simulink model "three_ringnetwork_with_control"  (R2016a)
settings: Solver=VariableStepAuto  StartTime=0.0  StopTime=0.2  RelTol=1e-3
undefined symbols (not defined in the file): vc0d
libraries: simulink x18, powerlib_meascontrol x3
(part 2 of 3)

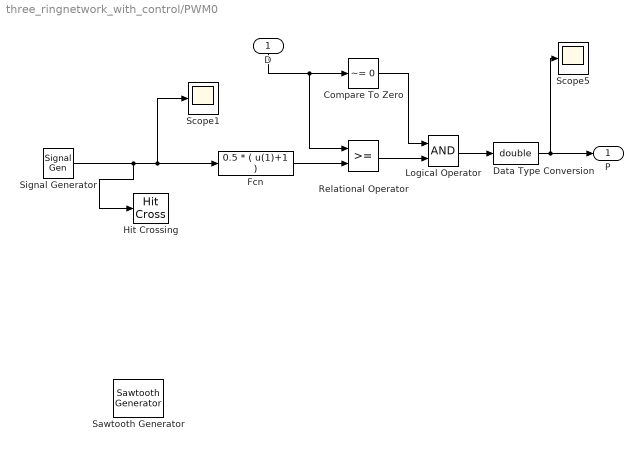
== system three_ringnetwork_with_control/PWM0 ==
  D : Inport
  Compare To Zero : simulink/Logic and Bit Operations/Compare To Zero  relop=~=  OutDataTypeStr=boolean
  Data Type Conversion : DataTypeConversion  OutMin=[0]  OutMax=[1]  OutDataTypeStr=double
  Fcn : Fcn  Expr=0.5 * ( u(1)+1 )
  Hit Crossing : HitCross  ShowOutputPort=off
  Logical Operator : Logic  AllPortsSameDT=off  OutDataTypeStr=boolean
  Relational Operator : RelationalOperator  OutDataTypeStr=boolean
  Sawtooth Generator : powerlib_meascontrol/Pulse & Signal Generators/Sawtooth Generator  Freq=1e3  Phase=180  Ts=0
  Scope1 : Scope
  Scope5 : Scope
  Signal Generator : SignalGenerator  WaveForm=sawtooth  Frequency=10000
  P : Outport
  wires:
  Logical Operator/1 -> Data Type Conversion/1
  Relational Operator/1 -> Logical Operator/2
  Fcn/1 -> Relational Operator/2
  D/1 -> Relational Operator/1, Compare To Zero/1
  Data Type Conversion/1 -> P/1, Scope5/1
  Compare To Zero/1 -> Logical Operator/1
  Signal Generator/1 -> Hit Crossing/1, Scope1/1, Fcn/1

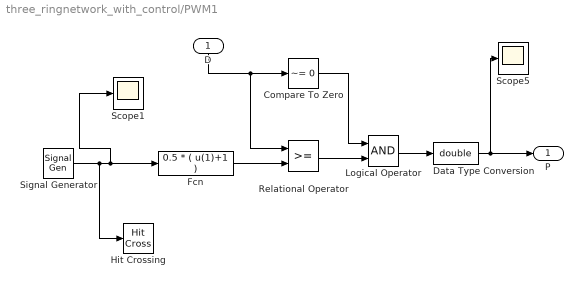
== system three_ringnetwork_with_control/PWM1 ==
  D : Inport
  Compare To Zero : simulink/Logic and Bit Operations/Compare To Zero  relop=~=  OutDataTypeStr=boolean
  Data Type Conversion : DataTypeConversion  OutDataTypeStr=double
  Fcn : Fcn  Expr=0.5 * ( u(1)+1 )
  Hit Crossing : HitCross
  Logical Operator : Logic  AllPortsSameDT=off  OutDataTypeStr=boolean
  Relational Operator : RelationalOperator  OutDataTypeStr=boolean
  Scope1 : Scope
  Scope5 : Scope
  Signal Generator : SignalGenerator  WaveForm=sawtooth  Frequency=10000
  P : Outport
  wires:
  Logical Operator/1 -> Data Type Conversion/1
  Relational Operator/1 -> Logical Operator/2
  Signal Generator/1 -> Hit Crossing/1, Scope1/1, Fcn/1
  Fcn/1 -> Relational Operator/2
  D/1 -> Relational Operator/1, Compare To Zero/1
  Data Type Conversion/1 -> P/1, Scope5/1
  Compare To Zero/1 -> Logical Operator/1

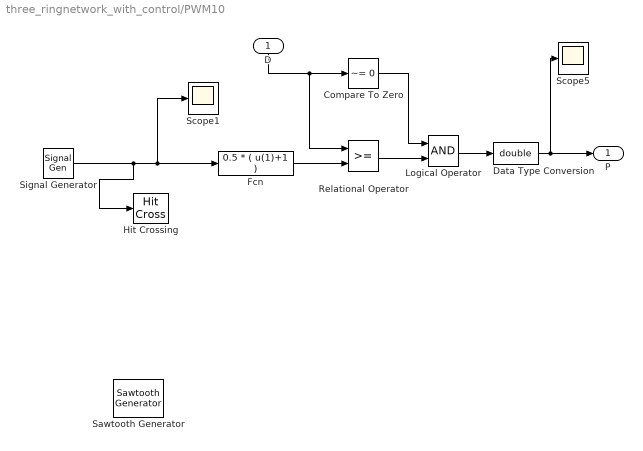
== system three_ringnetwork_with_control/PWM10 ==
  D : Inport
  Compare To Zero : simulink/Logic and Bit Operations/Compare To Zero  relop=~=  OutDataTypeStr=boolean  ZeroCross=off
  Data Type Conversion : DataTypeConversion  OutMin=[0]  OutMax=[1]  OutDataTypeStr=double
  Fcn : Fcn  Expr=0.5 * ( u(1)+1 )
  Hit Crossing : HitCross  ShowOutputPort=off
  Logical Operator : Logic  AllPortsSameDT=off  OutDataTypeStr=boolean
  Relational Operator : RelationalOperator  OutDataTypeStr=boolean  ZeroCross=off
  Sawtooth Generator : powerlib_meascontrol/Pulse & Signal Generators/Sawtooth Generator  Freq=1e3  Phase=180  Ts=0
  Scope1 : Scope
  Scope5 : Scope
  Signal Generator : SignalGenerator  WaveForm=sawtooth  Frequency=10000
  P : Outport
  wires:
  Logical Operator/1 -> Data Type Conversion/1
  Relational Operator/1 -> Logical Operator/2
  Fcn/1 -> Relational Operator/2
  D/1 -> Relational Operator/1, Compare To Zero/1
  Data Type Conversion/1 -> P/1, Scope5/1
  Compare To Zero/1 -> Logical Operator/1
  Signal Generator/1 -> Hit Crossing/1, Scope1/1, Fcn/1

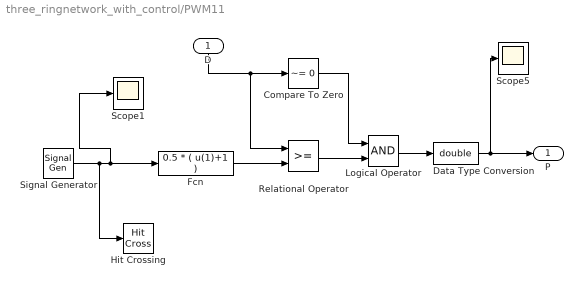
== system three_ringnetwork_with_control/PWM11 ==
  D : Inport
  Compare To Zero : simulink/Logic and Bit Operations/Compare To Zero  relop=~=  OutDataTypeStr=boolean
  Data Type Conversion : DataTypeConversion  OutDataTypeStr=double
  Fcn : Fcn  Expr=0.5 * ( u(1)+1 )
  Hit Crossing : HitCross
  Logical Operator : Logic  AllPortsSameDT=off  OutDataTypeStr=boolean
  Relational Operator : RelationalOperator  OutDataTypeStr=boolean
  Scope1 : Scope
  Scope5 : Scope
  Signal Generator : SignalGenerator  WaveForm=sawtooth  Frequency=10000
  P : Outport
  wires:
  Logical Operator/1 -> Data Type Conversion/1
  Relational Operator/1 -> Logical Operator/2
  Signal Generator/1 -> Hit Crossing/1, Scope1/1, Fcn/1
  Fcn/1 -> Relational Operator/2
  D/1 -> Relational Operator/1, Compare To Zero/1
  Data Type Conversion/1 -> P/1, Scope5/1
  Compare To Zero/1 -> Logical Operator/1

== system three_ringnetwork_with_control/PWM12 ==
  D : Inport
  Compare To Zero : simulink/Logic and Bit Operations/Compare To Zero  relop=~=  OutDataTypeStr=boolean
  Data Type Conversion : DataTypeConversion  OutDataTypeStr=double
  Fcn : Fcn  Expr=0.5 * ( u(1)+1 )
  Hit Crossing : HitCross
  Logical Operator : Logic  AllPortsSameDT=off  OutDataTypeStr=boolean
  Relational Operator : RelationalOperator  OutDataTypeStr=boolean
  Scope1 : Scope
  Scope5 : Scope
  Signal Generator : SignalGenerator  WaveForm=sawtooth  Frequency=10000
  P : Outport
  wires:
  Logical Operator/1 -> Data Type Conversion/1
  Relational Operator/1 -> Logical Operator/2
  Signal Generator/1 -> Hit Crossing/1, Scope1/1, Fcn/1
  Fcn/1 -> Relational Operator/2
  D/1 -> Relational Operator/1, Compare To Zero/1
  Data Type Conversion/1 -> P/1, Scope5/1
  Compare To Zero/1 -> Logical Operator/1

== system three_ringnetwork_with_control/PWM13 ==
  D : Inport
  Compare To Zero : simulink/Logic and Bit Operations/Compare To Zero  relop=~=  OutDataTypeStr=boolean
  Data Type Conversion : DataTypeConversion  OutDataTypeStr=double
  Fcn : Fcn  Expr=0.5 * ( u(1)+1 )
  Hit Crossing : HitCross
  Logical Operator : Logic  AllPortsSameDT=off  OutDataTypeStr=boolean
  Relational Operator : RelationalOperator  OutDataTypeStr=boolean
  Scope1 : Scope
  Scope5 : Scope
  Signal Generator : SignalGenerator  WaveForm=sawtooth  Frequency=10000
  P : Outport
  wires:
  Logical Operator/1 -> Data Type Conversion/1
  Relational Operator/1 -> Logical Operator/2
  Signal Generator/1 -> Scope1/1, Hit Crossing/1, Fcn/1
  Fcn/1 -> Relational Operator/2
  D/1 -> Relational Operator/1, Compare To Zero/1
  Data Type Conversion/1 -> P/1, Scope5/1
  Compare To Zero/1 -> Logical Operator/1

== system three_ringnetwork_with_control/PWM14 ==
  D : Inport
  Compare To Zero : simulink/Logic and Bit Operations/Compare To Zero  relop=~=  OutDataTypeStr=boolean
  Data Type Conversion : DataTypeConversion  OutDataTypeStr=double
  Fcn : Fcn  Expr=0.5 * ( u(1)+1 )
  Hit Crossing : HitCross
  Logical Operator : Logic  AllPortsSameDT=off  OutDataTypeStr=boolean
  Relational Operator : RelationalOperator  OutDataTypeStr=boolean
  Scope5 : Scope
  Signal Generator : SignalGenerator  WaveForm=sawtooth  Frequency=10000
  P : Outport
  wires:
  Logical Operator/1 -> Data Type Conversion/1
  Relational Operator/1 -> Logical Operator/2
  Signal Generator/1 -> Hit Crossing/1, Fcn/1
  Fcn/1 -> Relational Operator/2
  D/1 -> Relational Operator/1, Compare To Zero/1
  Data Type Conversion/1 -> P/1, Scope5/1
  Compare To Zero/1 -> Logical Operator/1

== system three_ringnetwork_with_control/PWM2 ==
  D : Inport
  Compare To Zero : simulink/Logic and Bit Operations/Compare To Zero  relop=~=  OutDataTypeStr=boolean
  Data Type Conversion : DataTypeConversion  OutDataTypeStr=double
  Fcn : Fcn  Expr=0.5 * ( u(1)+1 )
  Hit Crossing : HitCross
  Logical Operator : Logic  AllPortsSameDT=off  OutDataTypeStr=boolean
  Relational Operator : RelationalOperator  OutDataTypeStr=boolean
  Scope1 : Scope
  Scope5 : Scope
  Signal Generator : SignalGenerator  WaveForm=sawtooth  Frequency=10000
  P : Outport
  wires:
  Logical Operator/1 -> Data Type Conversion/1
  Relational Operator/1 -> Logical Operator/2
  Signal Generator/1 -> Hit Crossing/1, Scope1/1, Fcn/1
  Fcn/1 -> Relational Operator/2
  D/1 -> Relational Operator/1, Compare To Zero/1
  Data Type Conversion/1 -> P/1, Scope5/1
  Compare To Zero/1 -> Logical Operator/1

== system three_ringnetwork_with_control/PWM3 ==
  D : Inport
  Compare To Zero : simulink/Logic and Bit Operations/Compare To Zero  relop=~=  OutDataTypeStr=boolean
  Data Type Conversion : DataTypeConversion  OutDataTypeStr=double
  Fcn : Fcn  Expr=0.5 * ( u(1)+1 )
  Hit Crossing : HitCross
  Logical Operator : Logic  AllPortsSameDT=off  OutDataTypeStr=boolean
  Relational Operator : RelationalOperator  OutDataTypeStr=boolean
  Scope1 : Scope
  Scope5 : Scope
  Signal Generator : SignalGenerator  WaveForm=sawtooth  Frequency=10000
  P : Outport
  wires:
  Logical Operator/1 -> Data Type Conversion/1
  Relational Operator/1 -> Logical Operator/2
  Signal Generator/1 -> Scope1/1, Hit Crossing/1, Fcn/1
  Fcn/1 -> Relational Operator/2
  D/1 -> Relational Operator/1, Compare To Zero/1
  Data Type Conversion/1 -> P/1, Scope5/1
  Compare To Zero/1 -> Logical Operator/1

== system three_ringnetwork_with_control/PWM4 ==
  D : Inport
  Compare To Zero : simulink/Logic and Bit Operations/Compare To Zero  relop=~=  OutDataTypeStr=boolean
  Data Type Conversion : DataTypeConversion  OutDataTypeStr=double
  Fcn : Fcn  Expr=0.5 * ( u(1)+1 )
  Hit Crossing : HitCross
  Logical Operator : Logic  AllPortsSameDT=off  OutDataTypeStr=boolean
  Relational Operator : RelationalOperator  OutDataTypeStr=boolean
  Scope5 : Scope
  Signal Generator : SignalGenerator  WaveForm=sawtooth  Frequency=10000
  P : Outport
  wires:
  Logical Operator/1 -> Data Type Conversion/1
  Relational Operator/1 -> Logical Operator/2
  Signal Generator/1 -> Hit Crossing/1, Fcn/1
  Fcn/1 -> Relational Operator/2
  D/1 -> Relational Operator/1, Compare To Zero/1
  Data Type Conversion/1 -> P/1, Scope5/1
  Compare To Zero/1 -> Logical Operator/1

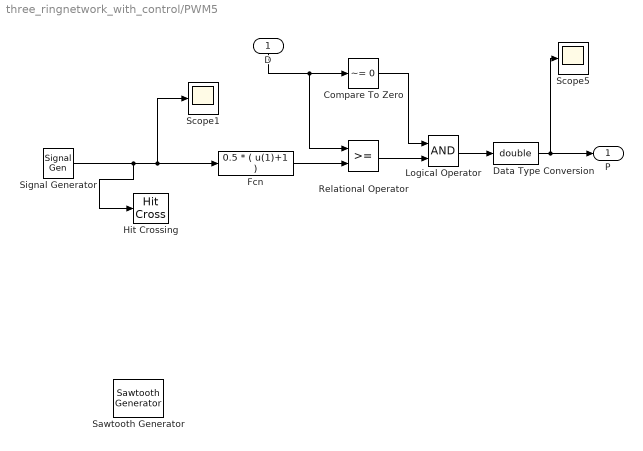
== system three_ringnetwork_with_control/PWM5 ==
  D : Inport
  Compare To Zero : simulink/Logic and Bit Operations/Compare To Zero  relop=~=  OutDataTypeStr=boolean
  Data Type Conversion : DataTypeConversion  OutMin=[0]  OutMax=[1]  OutDataTypeStr=double
  Fcn : Fcn  Expr=0.5 * ( u(1)+1 )
  Hit Crossing : HitCross  ShowOutputPort=off
  Logical Operator : Logic  AllPortsSameDT=off  OutDataTypeStr=boolean
  Relational Operator : RelationalOperator  OutDataTypeStr=boolean
  Sawtooth Generator : powerlib_meascontrol/Pulse & Signal Generators/Sawtooth Generator  Freq=1e3  Phase=180  Ts=0
  Scope1 : Scope
  Scope5 : Scope
  Signal Generator : SignalGenerator  WaveForm=sawtooth  Frequency=10000
  P : Outport
  wires:
  Logical Operator/1 -> Data Type Conversion/1
  Relational Operator/1 -> Logical Operator/2
  Fcn/1 -> Relational Operator/2
  D/1 -> Relational Operator/1, Compare To Zero/1
  Data Type Conversion/1 -> P/1, Scope5/1
  Compare To Zero/1 -> Logical Operator/1
  Signal Generator/1 -> Hit Crossing/1, Scope1/1, Fcn/1

== system three_ringnetwork_with_control/PWM6 ==
  D : Inport
  Compare To Zero : simulink/Logic and Bit Operations/Compare To Zero  relop=~=  OutDataTypeStr=boolean
  Data Type Conversion : DataTypeConversion  OutDataTypeStr=double
  Fcn : Fcn  Expr=0.5 * ( u(1)+1 )
  Hit Crossing : HitCross
  Logical Operator : Logic  AllPortsSameDT=off  OutDataTypeStr=boolean
  Relational Operator : RelationalOperator  OutDataTypeStr=boolean
  Scope1 : Scope
  Scope5 : Scope
  Signal Generator : SignalGenerator  WaveForm=sawtooth  Frequency=10000
  P : Outport
  wires:
  Logical Operator/1 -> Data Type Conversion/1
  Relational Operator/1 -> Logical Operator/2
  Signal Generator/1 -> Hit Crossing/1, Scope1/1, Fcn/1
  Fcn/1 -> Relational Operator/2
  D/1 -> Relational Operator/1, Compare To Zero/1
  Data Type Conversion/1 -> P/1, Scope5/1
  Compare To Zero/1 -> Logical Operator/1

== system three_ringnetwork_with_control/PWM7 ==
  D : Inport
  Compare To Zero : simulink/Logic and Bit Operations/Compare To Zero  relop=~=  OutDataTypeStr=boolean
  Data Type Conversion : DataTypeConversion  OutDataTypeStr=double
  Fcn : Fcn  Expr=0.5 * ( u(1)+1 )
  Hit Crossing : HitCross
  Logical Operator : Logic  AllPortsSameDT=off  OutDataTypeStr=boolean
  Relational Operator : RelationalOperator  OutDataTypeStr=boolean
  Scope1 : Scope
  Scope5 : Scope
  Signal Generator : SignalGenerator  WaveForm=sawtooth  Frequency=10000
  P : Outport
  wires:
  Logical Operator/1 -> Data Type Conversion/1
  Relational Operator/1 -> Logical Operator/2
  Signal Generator/1 -> Hit Crossing/1, Scope1/1, Fcn/1
  Fcn/1 -> Relational Operator/2
  D/1 -> Relational Operator/1, Compare To Zero/1
  Data Type Conversion/1 -> P/1, Scope5/1
  Compare To Zero/1 -> Logical Operator/1

== system three_ringnetwork_with_control/PWM8 ==
  D : Inport
  Compare To Zero : simulink/Logic and Bit Operations/Compare To Zero  relop=~=  OutDataTypeStr=boolean
  Data Type Conversion : DataTypeConversion  OutDataTypeStr=double
  Fcn : Fcn  Expr=0.5 * ( u(1)+1 )
  Hit Crossing : HitCross
  Logical Operator : Logic  AllPortsSameDT=off  OutDataTypeStr=boolean
  Relational Operator : RelationalOperator  OutDataTypeStr=boolean
  Scope1 : Scope
  Scope5 : Scope
  Signal Generator : SignalGenerator  WaveForm=sawtooth  Frequency=10000
  P : Outport
  wires:
  Logical Operator/1 -> Data Type Conversion/1
  Relational Operator/1 -> Logical Operator/2
  Signal Generator/1 -> Scope1/1, Hit Crossing/1, Fcn/1
  Fcn/1 -> Relational Operator/2
  D/1 -> Relational Operator/1, Compare To Zero/1
  Data Type Conversion/1 -> P/1, Scope5/1
  Compare To Zero/1 -> Logical Operator/1

== system three_ringnetwork_with_control/PWM9 ==
  D : Inport
  Compare To Zero : simulink/Logic and Bit Operations/Compare To Zero  relop=~=  OutDataTypeStr=boolean
  Data Type Conversion : DataTypeConversion  OutDataTypeStr=double
  Fcn : Fcn  Expr=0.5 * ( u(1)+1 )
  Hit Crossing : HitCross
  Logical Operator : Logic  AllPortsSameDT=off  OutDataTypeStr=boolean
  Relational Operator : RelationalOperator  OutDataTypeStr=boolean
  Scope5 : Scope
  Signal Generator : SignalGenerator  WaveForm=sawtooth  Frequency=10000
  P : Outport
  wires:
  Logical Operator/1 -> Data Type Conversion/1
  Relational Operator/1 -> Logical Operator/2
  Signal Generator/1 -> Hit Crossing/1, Fcn/1
  Fcn/1 -> Relational Operator/2
  D/1 -> Relational Operator/1, Compare To Zero/1
  Data Type Conversion/1 -> P/1, Scope5/1
  Compare To Zero/1 -> Logical Operator/1

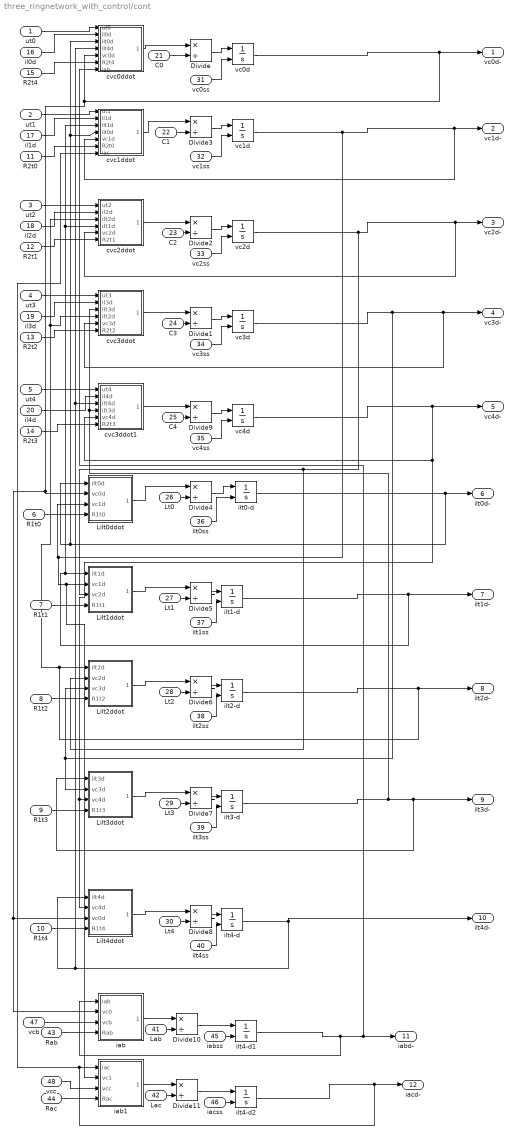
== system three_ringnetwork_with_control/cont ==
  ut0 : Inport
  ut1 : Inport  Port=2
  ut2 : Inport  Port=3
  ut3 : Inport  Port=4
  ut4 : Inport  Port=5
  R1t0 : Inport  Port=6
  R1t1 : Inport  Port=7
  R1t2 : Inport  Port=8
  R1t3 : Inport  Port=9
  R1t4 : Inport  Port=10
  R2t0 : Inport  Port=11
  R2t1 : Inport  Port=12
  R2t2 : Inport  Port=13
  R2t3 : Inport  Port=14
  R2t4 : Inport  Port=15
  il0d : Inport  Port=16
  il1d : Inport  Port=17
  il2d : Inport  Port=18
  il3d : Inport  Port=19
  il4d : Inport  Port=20
  C0 : Inport  Port=21
  C1 : Inport  Port=22
  C2 : Inport  Port=23
  C3 : Inport  Port=24
  C4 : Inport  Port=25
  Lt0 : Inport  Port=26
  Lt1 : Inport  Port=27
  Lt2 : Inport  Port=28
  Lt3 : Inport  Port=29
  Lt4 : Inport  Port=30
  vc0ss : Inport  Port=31
  vc1ss : Inport  Port=32
  vc2ss : Inport  Port=33
  vc3ss : Inport  Port=34
  vc4ss : Inport  Port=35
  ilt0ss : Inport  Port=36
  ilt1ss : Inport  Port=37
  ilt2ss : Inport  Port=38
  ilt3ss : Inport  Port=39
  ilt4ss : Inport  Port=40
  Lab : Inport  Port=41
  Lac : Inport  Port=42
  Rab : Inport  Port=43
  Rac : Inport  Port=44
  iabss : Inport  Port=45
  iacss : Inport  Port=46
  vcb : Inport  Port=47
  vcc : Inport  Port=48
  Divide{,1..11} (12 alike) : Product  Inputs=*/
  Lilt0ddot : MATLAB Function  TreatAsAtomicUnit=on
  Lilt1ddot : MATLAB Function  TreatAsAtomicUnit=on
  Lilt2ddot : MATLAB Function  TreatAsAtomicUnit=on
  Lilt3ddot : MATLAB Function  TreatAsAtomicUnit=on
  Lilt4ddot : MATLAB Function  TreatAsAtomicUnit=on
  cvc0ddot : MATLAB Function  TreatAsAtomicUnit=on
  cvc1ddot : MATLAB Function  TreatAsAtomicUnit=on
  cvc2ddot : MATLAB Function  TreatAsAtomicUnit=on
  cvc3ddot : MATLAB Function  TreatAsAtomicUnit=on
  cvc3ddot1 : MATLAB Function  TreatAsAtomicUnit=on
  iab : MATLAB Function  TreatAsAtomicUnit=on
  iab1 : MATLAB Function  TreatAsAtomicUnit=on
  ilt0-d : Integrator  InitialConditionSource=external  InitialCondition=vc0d
  ilt1-d : Integrator  InitialConditionSource=external  InitialCondition=vc0d
  ilt2-d : Integrator  InitialConditionSource=external  InitialCondition=vc0d
  ilt3-d : Integrator  InitialConditionSource=external  InitialCondition=vc0d
  ilt4-d : Integrator  InitialConditionSource=external  InitialCondition=vc0d
  ilt4-d1 : Integrator  InitialConditionSource=external  InitialCondition=vc0d
  ilt4-d2 : Integrator  InitialConditionSource=external  InitialCondition=vc0d
  vc0d : Integrator  InitialConditionSource=external  InitialCondition=vc0d
  vc1d : Integrator  InitialConditionSource=external  InitialCondition=vc0d
  vc2d : Integrator  InitialConditionSource=external  InitialCondition=vc0d
  vc3d : Integrator  InitialConditionSource=external  InitialCondition=vc0d
  vc4d : Integrator  InitialConditionSource=external  InitialCondition=vc0d
  vc0d- : Outport
  vc1d- : Outport  Port=2
  vc2d- : Outport  Port=3
  vc3d- : Outport  Port=4
  vc4d- : Outport  Port=5
  ilt0d- : Outport  Port=6
  ilt1d- : Outport  Port=7
  ilt2d- : Outport  Port=8
  ilt3d- : Outport  Port=9
  ilt4d- : Outport  Port=10
  iabd- : Outport  Port=11
  iacd- : Outport  Port=12
  wires:
  cvc0ddot/1(Cvc0ddot) -> Divide/1
  ut0/1 -> cvc0ddot/1(ut0)
  il0d/1 -> cvc0ddot/2(il0d)
  C0/1 -> Divide/2
  C1/1 -> Divide3/2
  C2/1 -> Divide2/2
  Divide3/1 -> vc1d/1
  Divide/1 -> vc0d/1
  cvc1ddot/1(Cvc1ddot) -> Divide3/1
  ut1/1 -> cvc1ddot/1(ut1)
  il1d/1 -> cvc1ddot/2(il1d)
  R2t4/1 -> cvc0ddot/6(R2t4)
  R2t0/1 -> cvc1ddot/6(R2t0)
  cvc2ddot/1(Cvc2ddot) -> Divide2/1
  ut2/1 -> cvc2ddot/1(ut2)
  il2d/1 -> cvc2ddot/2(il2d)
  R2t1/1 -> cvc2ddot/6(R2t1)
  Divide2/1 -> vc2d/1
  Divide4/1 -> ilt0-d/1
  Divide5/1 -> ilt1-d/1
  Divide6/1 -> ilt2-d/1
  Lt0/1 -> Divide4/2
  Lt1/1 -> Divide5/2
  Lt2/1 -> Divide6/2
  Lilt2ddot/1(Lilt2ddot) -> Divide6/1
  Lilt1ddot/1(Lilt1ddot) -> Divide5/1
  Lilt0ddot/1(Lilt0ddot) -> Divide4/1
  R1t1/1 -> Lilt1ddot/4(R1t1)
  R1t2/1 -> Lilt2ddot/4(R1t2)
  vc0ss/1 -> vc0d/2
  vc1ss/1 -> vc1d/2
  vc2ss/1 -> vc2d/2
  ilt0ss/1 -> ilt0-d/2
  ilt2ss/1 -> ilt2-d/2
  ilt1ss/1 -> ilt1-d/2
  R1t0/1 -> Lilt0ddot/4(R1t0)
  C3/1 -> Divide1/2
  cvc3ddot/1(Cvc3ddot) -> Divide1/1
  ut3/1 -> cvc3ddot/1(ut3)
  il3d/1 -> cvc3ddot/2(il3d)
  R2t2/1 -> cvc3ddot/6(R2t2)
  Divide1/1 -> vc3d/1
  vc3ss/1 -> vc3d/2
  Divide7/1 -> ilt3-d/1
  Lt3/1 -> Divide7/2
  Lilt3ddot/1(Lilt3ddot) -> Divide7/1
  R1t3/1 -> Lilt3ddot/4(R1t3)
  ilt3ss/1 -> ilt3-d/2
  Divide8/1 -> ilt4-d/1
  Lt4/1 -> Divide8/2
  Lilt4ddot/1(Lilt4ddot) -> Divide8/1
  R1t4/1 -> Lilt4ddot/4(R1t4)
  ilt4ss/1 -> ilt4-d/2
  C4/1 -> Divide9/2
  cvc3ddot1/1(Cvc4ddot) -> Divide9/1
  Divide9/1 -> vc4d/1
  vc4ss/1 -> vc4d/2
  vc0d/1 -> cvc0ddot/5(vc0d), iab/2(vc0), Lilt4ddot/3(vc0d), Lilt0ddot/2(vc0d), vc0d-/1
  vc1d/1 -> iab1/2(vc1), Lilt1ddot/2(vc1d), Lilt0ddot/3(vc1d), cvc1ddot/5(vc1d), vc1d-/1
  vc2d/1 -> Lilt2ddot/2(vc2d), Lilt1ddot/3(vc2d), cvc2ddot/5(vc2d), vc2d-/1
  vc3d/1 -> Lilt3ddot/2(vc3d), Lilt2ddot/3(vc3d), cvc3ddot/5(vc3d), vc3d-/1
  vc4d/1 -> cvc3ddot1/5(vc4d), Lilt4ddot/2(vc4d), Lilt3ddot/3(vc4d), vc4d-/1
  ilt0-d/1 -> cvc0ddot/3(ilt0d), cvc1ddot/4(ilt0d), Lilt0ddot/1(ilt0d), ilt0d-/1
  ilt1-d/1 -> cvc2ddot/4(ilt1d), cvc1ddot/3(ilt1d), Lilt1ddot/1(ilt1d), ilt1d-/1
  ilt2-d/1 -> Lilt2ddot/1(ilt2d), cvc3ddot/4(ilt2d), cvc2ddot/3(ilt2d), ilt2d-/1
  ilt4-d/1 -> cvc0ddot/4(ilt4d), cvc3ddot1/3(ilt4d), Lilt4ddot/1(ilt4d), ilt4d-/1
  ut4/1 -> cvc3ddot1/1(ut4)
  il4d/1 -> cvc3ddot1/2(il4d)
  R2t3/1 -> cvc3ddot1/6(R2t3)
  ilt3-d/1 -> cvc3ddot/3(ilt3d), cvc3ddot1/4(ilt3d), Lilt3ddot/1(ilt3d), ilt3d-/1
  iab/1(Labddot) -> Divide10/1
  Divide10/1 -> ilt4-d1/1
  iab1/1(Lacddot) -> Divide11/1
  Divide11/1 -> ilt4-d2/1
  ilt4-d1/1 -> iab/1(iab), cvc0ddot/7(iab), iabd-/1
  ilt4-d2/1 -> cvc1ddot/7(iac), iab1/1(iac), iacd-/1
  Lab/1 -> Divide10/2
  Lac/1 -> Divide11/2
  Rac/1 -> iab1/4(Rac)
  Rab/1 -> iab/4(Rab)
  iabss/1 -> ilt4-d1/2
  iacss/1 -> ilt4-d2/2
  vcb/1 -> iab/3(vcb)
  vcc/1 -> iab1/3(vcc)

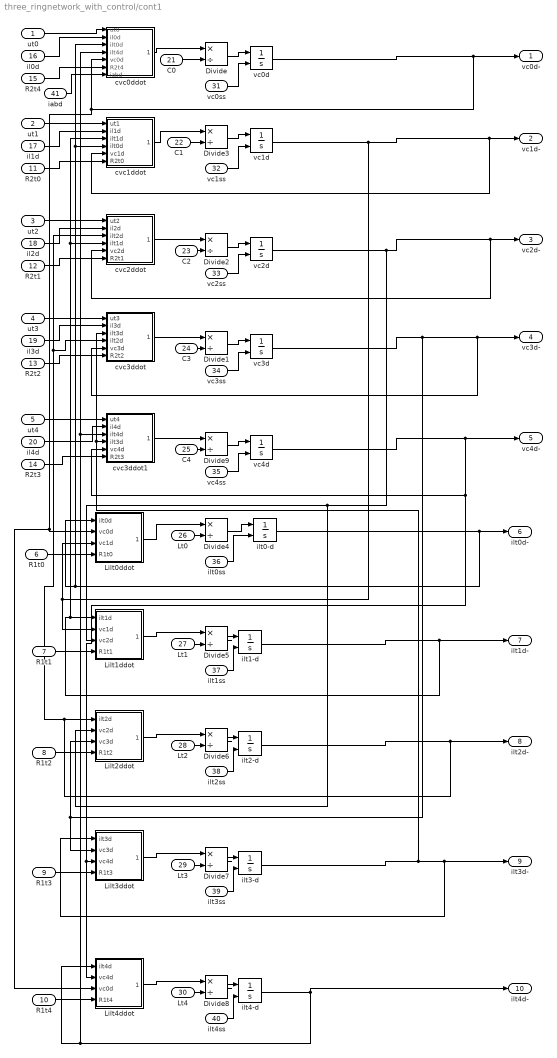
== system three_ringnetwork_with_control/cont1 ==
  ut0 : Inport
  ut1 : Inport  Port=2
  ut2 : Inport  Port=3
  ut3 : Inport  Port=4
  ut4 : Inport  Port=5
  R1t0 : Inport  Port=6
  R1t1 : Inport  Port=7
  R1t2 : Inport  Port=8
  R1t3 : Inport  Port=9
  R1t4 : Inport  Port=10
  R2t0 : Inport  Port=11
  R2t1 : Inport  Port=12
  R2t2 : Inport  Port=13
  R2t3 : Inport  Port=14
  R2t4 : Inport  Port=15
  il0d : Inport  Port=16
  il1d : Inport  Port=17
  il2d : Inport  Port=18
  il3d : Inport  Port=19
  il4d : Inport  Port=20
  C0 : Inport  Port=21
  C1 : Inport  Port=22
  C2 : Inport  Port=23
  C3 : Inport  Port=24
  C4 : Inport  Port=25
  Lt0 : Inport  Port=26
  Lt1 : Inport  Port=27
  Lt2 : Inport  Port=28
  Lt3 : Inport  Port=29
  Lt4 : Inport  Port=30
  vc0ss : Inport  Port=31
  vc1ss : Inport  Port=32
  vc2ss : Inport  Port=33
  vc3ss : Inport  Port=34
  vc4ss : Inport  Port=35
  ilt0ss : Inport  Port=36
  ilt1ss : Inport  Port=37
  ilt2ss : Inport  Port=38
  ilt3ss : Inport  Port=39
  ilt4ss : Inport  Port=40
  iabd : Inport  Port=41
  Divide{,1..9} (10 alike) : Product  Inputs=*/
  Lilt0ddot : MATLAB Function  TreatAsAtomicUnit=on
  Lilt1ddot : MATLAB Function  TreatAsAtomicUnit=on
  Lilt2ddot : MATLAB Function  TreatAsAtomicUnit=on
  Lilt3ddot : MATLAB Function  TreatAsAtomicUnit=on
  Lilt4ddot : MATLAB Function  TreatAsAtomicUnit=on
  cvc0ddot : MATLAB Function  TreatAsAtomicUnit=on
  cvc1ddot : MATLAB Function  TreatAsAtomicUnit=on
  cvc2ddot : MATLAB Function  TreatAsAtomicUnit=on
  cvc3ddot : MATLAB Function  TreatAsAtomicUnit=on
  cvc3ddot1 : MATLAB Function  TreatAsAtomicUnit=on
  ilt0-d : Integrator  InitialConditionSource=external  InitialCondition=vc0d
  ilt1-d : Integrator  InitialConditionSource=external  InitialCondition=vc0d
  ilt2-d : Integrator  InitialConditionSource=external  InitialCondition=vc0d
  ilt3-d : Integrator  InitialConditionSource=external  InitialCondition=vc0d
  ilt4-d : Integrator  InitialConditionSource=external  InitialCondition=vc0d
  vc0d : Integrator  InitialConditionSource=external  InitialCondition=vc0d
  vc1d : Integrator  InitialConditionSource=external  InitialCondition=vc0d
  vc2d : Integrator  InitialConditionSource=external  InitialCondition=vc0d
  vc3d : Integrator  InitialConditionSource=external  InitialCondition=vc0d
  vc4d : Integrator  InitialConditionSource=external  InitialCondition=vc0d
  vc0d- : Outport
  vc1d- : Outport  Port=2
  vc2d- : Outport  Port=3
  vc3d- : Outport  Port=4
  vc4d- : Outport  Port=5
  ilt0d- : Outport  Port=6
  ilt1d- : Outport  Port=7
  ilt2d- : Outport  Port=8
  ilt3d- : Outport  Port=9
  ilt4d- : Outport  Port=10
  wires:
  cvc0ddot/1(Cvc0ddot) -> Divide/1
  ut0/1 -> cvc0ddot/1(ut0)
  il0d/1 -> cvc0ddot/2(il0d)
  C0/1 -> Divide/2
  C1/1 -> Divide3/2
  C2/1 -> Divide2/2
  Divide3/1 -> vc1d/1
  Divide/1 -> vc0d/1
  cvc1ddot/1(Cvc1ddot) -> Divide3/1
  ut1/1 -> cvc1ddot/1(ut1)
  il1d/1 -> cvc1ddot/2(il1d)
  R2t4/1 -> cvc0ddot/6(R2t4)
  R2t0/1 -> cvc1ddot/6(R2t0)
  cvc2ddot/1(Cvc2ddot) -> Divide2/1
  ut2/1 -> cvc2ddot/1(ut2)
  il2d/1 -> cvc2ddot/2(il2d)
  R2t1/1 -> cvc2ddot/6(R2t1)
  Divide2/1 -> vc2d/1
  Divide4/1 -> ilt0-d/1
  Divide5/1 -> ilt1-d/1
  Divide6/1 -> ilt2-d/1
  Lt0/1 -> Divide4/2
  Lt1/1 -> Divide5/2
  Lt2/1 -> Divide6/2
  Lilt2ddot/1(Lilt2ddot) -> Divide6/1
  Lilt1ddot/1(Lilt1ddot) -> Divide5/1
  Lilt0ddot/1(Lilt0ddot) -> Divide4/1
  R1t1/1 -> Lilt1ddot/4(R1t1)
  R1t2/1 -> Lilt2ddot/4(R1t2)
  vc0ss/1 -> vc0d/2
  vc1ss/1 -> vc1d/2
  vc2ss/1 -> vc2d/2
  ilt0ss/1 -> ilt0-d/2
  ilt2ss/1 -> ilt2-d/2
  ilt1ss/1 -> ilt1-d/2
  R1t0/1 -> Lilt0ddot/4(R1t0)
  C3/1 -> Divide1/2
  cvc3ddot/1(Cvc3ddot) -> Divide1/1
  ut3/1 -> cvc3ddot/1(ut3)
  il3d/1 -> cvc3ddot/2(il3d)
  R2t2/1 -> cvc3ddot/6(R2t2)
  Divide1/1 -> vc3d/1
  vc3ss/1 -> vc3d/2
  Divide7/1 -> ilt3-d/1
  Lt3/1 -> Divide7/2
  Lilt3ddot/1(Lilt3ddot) -> Divide7/1
  R1t3/1 -> Lilt3ddot/4(R1t3)
  ilt3ss/1 -> ilt3-d/2
  Divide8/1 -> ilt4-d/1
  Lt4/1 -> Divide8/2
  Lilt4ddot/1(Lilt4ddot) -> Divide8/1
  R1t4/1 -> Lilt4ddot/4(R1t4)
  ilt4ss/1 -> ilt4-d/2
  C4/1 -> Divide9/2
  cvc3ddot1/1(Cvc4ddot) -> Divide9/1
  Divide9/1 -> vc4d/1
  vc4ss/1 -> vc4d/2
  vc0d/1 -> cvc0ddot/5(vc0d), Lilt4ddot/3(vc0d), Lilt0ddot/2(vc0d), vc0d-/1
  vc1d/1 -> Lilt1ddot/2(vc1d), Lilt0ddot/3(vc1d), cvc1ddot/5(vc1d), vc1d-/1
  vc2d/1 -> Lilt2ddot/2(vc2d), Lilt1ddot/3(vc2d), cvc2ddot/5(vc2d), vc2d-/1
  vc3d/1 -> Lilt3ddot/2(vc3d), Lilt2ddot/3(vc3d), cvc3ddot/5(vc3d), vc3d-/1
  vc4d/1 -> cvc3ddot1/5(vc4d), Lilt4ddot/2(vc4d), Lilt3ddot/3(vc4d), vc4d-/1
  ilt0-d/1 -> cvc0ddot/3(ilt0d), cvc1ddot/4(ilt0d), Lilt0ddot/1(ilt0d), ilt0d-/1
  ilt1-d/1 -> cvc2ddot/4(ilt1d), cvc1ddot/3(ilt1d), Lilt1ddot/1(ilt1d), ilt1d-/1
  ilt2-d/1 -> Lilt2ddot/1(ilt2d), cvc3ddot/4(ilt2d), cvc2ddot/3(ilt2d), ilt2d-/1
  ilt4-d/1 -> cvc0ddot/4(ilt4d), cvc3ddot1/3(ilt4d), Lilt4ddot/1(ilt4d), ilt4d-/1
  ut4/1 -> cvc3ddot1/1(ut4)
  il4d/1 -> cvc3ddot1/2(il4d)
  R2t3/1 -> cvc3ddot1/6(R2t3)
  ilt3-d/1 -> cvc3ddot/3(ilt3d), cvc3ddot1/4(ilt3d), Lilt3ddot/1(ilt3d), ilt3d-/1
  iabd/1 -> cvc0ddot/7(iabd)

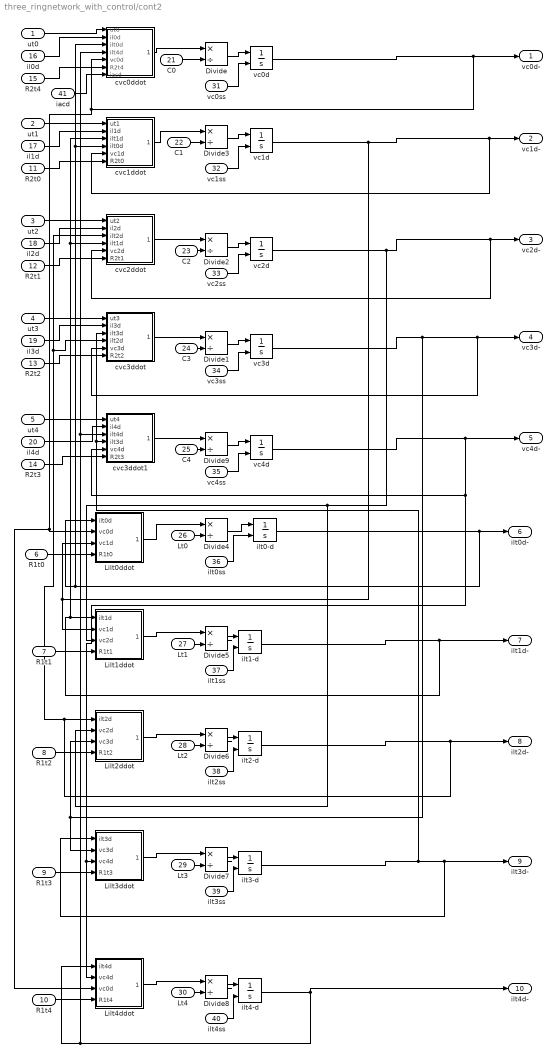
== system three_ringnetwork_with_control/cont2 ==
  ut0 : Inport
  ut1 : Inport  Port=2
  ut2 : Inport  Port=3
  ut3 : Inport  Port=4
  ut4 : Inport  Port=5
  R1t0 : Inport  Port=6
  R1t1 : Inport  Port=7
  R1t2 : Inport  Port=8
  R1t3 : Inport  Port=9
  R1t4 : Inport  Port=10
  R2t0 : Inport  Port=11
  R2t1 : Inport  Port=12
  R2t2 : Inport  Port=13
  R2t3 : Inport  Port=14
  R2t4 : Inport  Port=15
  il0d : Inport  Port=16
  il1d : Inport  Port=17
  il2d : Inport  Port=18
  il3d : Inport  Port=19
  il4d : Inport  Port=20
  C0 : Inport  Port=21
  C1 : Inport  Port=22
  C2 : Inport  Port=23
  C3 : Inport  Port=24
  C4 : Inport  Port=25
  Lt0 : Inport  Port=26
  Lt1 : Inport  Port=27
  Lt2 : Inport  Port=28
  Lt3 : Inport  Port=29
  Lt4 : Inport  Port=30
  vc0ss : Inport  Port=31
  vc1ss : Inport  Port=32
  vc2ss : Inport  Port=33
  vc3ss : Inport  Port=34
  vc4ss : Inport  Port=35
  ilt0ss : Inport  Port=36
  ilt1ss : Inport  Port=37
  ilt2ss : Inport  Port=38
  ilt3ss : Inport  Port=39
  ilt4ss : Inport  Port=40
  iacd : Inport  Port=41
  Divide{,1..9} (10 alike) : Product  Inputs=*/
  Lilt0ddot : MATLAB Function  TreatAsAtomicUnit=on
  Lilt1ddot : MATLAB Function  TreatAsAtomicUnit=on
  Lilt2ddot : MATLAB Function  TreatAsAtomicUnit=on
  Lilt3ddot : MATLAB Function  TreatAsAtomicUnit=on
  Lilt4ddot : MATLAB Function  TreatAsAtomicUnit=on
  cvc0ddot : MATLAB Function  TreatAsAtomicUnit=on
  cvc1ddot : MATLAB Function  TreatAsAtomicUnit=on
  cvc2ddot : MATLAB Function  TreatAsAtomicUnit=on
  cvc3ddot : MATLAB Function  TreatAsAtomicUnit=on
  cvc3ddot1 : MATLAB Function  TreatAsAtomicUnit=on
  ilt0-d : Integrator  InitialConditionSource=external  InitialCondition=vc0d
  ilt1-d : Integrator  InitialConditionSource=external  InitialCondition=vc0d
  ilt2-d : Integrator  InitialConditionSource=external  InitialCondition=vc0d
  ilt3-d : Integrator  InitialConditionSource=external  InitialCondition=vc0d
  ilt4-d : Integrator  InitialConditionSource=external  InitialCondition=vc0d
  vc0d : Integrator  InitialConditionSource=external  InitialCondition=vc0d
  vc1d : Integrator  InitialConditionSource=external  InitialCondition=vc0d
  vc2d : Integrator  InitialConditionSource=external  InitialCondition=vc0d
  vc3d : Integrator  InitialConditionSource=external  InitialCondition=vc0d
  vc4d : Integrator  InitialConditionSource=external  InitialCondition=vc0d
  vc0d- : Outport
  vc1d- : Outport  Port=2
  vc2d- : Outport  Port=3
  vc3d- : Outport  Port=4
  vc4d- : Outport  Port=5
  ilt0d- : Outport  Port=6
  ilt1d- : Outport  Port=7
  ilt2d- : Outport  Port=8
  ilt3d- : Outport  Port=9
  ilt4d- : Outport  Port=10
  wires:
  cvc0ddot/1(Cvc0ddot) -> Divide/1
  ut0/1 -> cvc0ddot/1(ut0)
  il0d/1 -> cvc0ddot/2(il0d)
  C0/1 -> Divide/2
  C1/1 -> Divide3/2
  C2/1 -> Divide2/2
  Divide3/1 -> vc1d/1
  Divide/1 -> vc0d/1
  cvc1ddot/1(Cvc1ddot) -> Divide3/1
  ut1/1 -> cvc1ddot/1(ut1)
  il1d/1 -> cvc1ddot/2(il1d)
  R2t4/1 -> cvc0ddot/6(R2t4)
  R2t0/1 -> cvc1ddot/6(R2t0)
  cvc2ddot/1(Cvc2ddot) -> Divide2/1
  ut2/1 -> cvc2ddot/1(ut2)
  il2d/1 -> cvc2ddot/2(il2d)
  R2t1/1 -> cvc2ddot/6(R2t1)
  Divide2/1 -> vc2d/1
  Divide4/1 -> ilt0-d/1
  Divide5/1 -> ilt1-d/1
  Divide6/1 -> ilt2-d/1
  Lt0/1 -> Divide4/2
  Lt1/1 -> Divide5/2
  Lt2/1 -> Divide6/2
  Lilt2ddot/1(Lilt2ddot) -> Divide6/1
  Lilt1ddot/1(Lilt1ddot) -> Divide5/1
  Lilt0ddot/1(Lilt0ddot) -> Divide4/1
  R1t1/1 -> Lilt1ddot/4(R1t1)
  R1t2/1 -> Lilt2ddot/4(R1t2)
  vc0ss/1 -> vc0d/2
  vc1ss/1 -> vc1d/2
  vc2ss/1 -> vc2d/2
  ilt0ss/1 -> ilt0-d/2
  ilt2ss/1 -> ilt2-d/2
  ilt1ss/1 -> ilt1-d/2
  R1t0/1 -> Lilt0ddot/4(R1t0)
  C3/1 -> Divide1/2
  cvc3ddot/1(Cvc3ddot) -> Divide1/1
  ut3/1 -> cvc3ddot/1(ut3)
  il3d/1 -> cvc3ddot/2(il3d)
  R2t2/1 -> cvc3ddot/6(R2t2)
  Divide1/1 -> vc3d/1
  vc3ss/1 -> vc3d/2
  Divide7/1 -> ilt3-d/1
  Lt3/1 -> Divide7/2
  Lilt3ddot/1(Lilt3ddot) -> Divide7/1
  R1t3/1 -> Lilt3ddot/4(R1t3)
  ilt3ss/1 -> ilt3-d/2
  Divide8/1 -> ilt4-d/1
  Lt4/1 -> Divide8/2
  Lilt4ddot/1(Lilt4ddot) -> Divide8/1
  R1t4/1 -> Lilt4ddot/4(R1t4)
  ilt4ss/1 -> ilt4-d/2
  C4/1 -> Divide9/2
  cvc3ddot1/1(Cvc4ddot) -> Divide9/1
  Divide9/1 -> vc4d/1
  vc4ss/1 -> vc4d/2
  vc0d/1 -> cvc0ddot/5(vc0d), Lilt4ddot/3(vc0d), Lilt0ddot/2(vc0d), vc0d-/1
  vc1d/1 -> Lilt1ddot/2(vc1d), Lilt0ddot/3(vc1d), cvc1ddot/5(vc1d), vc1d-/1
  vc2d/1 -> Lilt2ddot/2(vc2d), Lilt1ddot/3(vc2d), cvc2ddot/5(vc2d), vc2d-/1
  vc3d/1 -> Lilt3ddot/2(vc3d), Lilt2ddot/3(vc3d), cvc3ddot/5(vc3d), vc3d-/1
  vc4d/1 -> cvc3ddot1/5(vc4d), Lilt4ddot/2(vc4d), Lilt3ddot/3(vc4d), vc4d-/1
  ilt0-d/1 -> cvc0ddot/3(ilt0d), cvc1ddot/4(ilt0d), Lilt0ddot/1(ilt0d), ilt0d-/1
  ilt1-d/1 -> cvc2ddot/4(ilt1d), cvc1ddot/3(ilt1d), Lilt1ddot/1(ilt1d), ilt1d-/1
  ilt2-d/1 -> Lilt2ddot/1(ilt2d), cvc3ddot/4(ilt2d), cvc2ddot/3(ilt2d), ilt2d-/1
  ilt4-d/1 -> cvc0ddot/4(ilt4d), cvc3ddot1/3(ilt4d), Lilt4ddot/1(ilt4d), ilt4d-/1
  ut4/1 -> cvc3ddot1/1(ut4)
  il4d/1 -> cvc3ddot1/2(il4d)
  R2t3/1 -> cvc3ddot1/6(R2t3)
  ilt3-d/1 -> cvc3ddot/3(ilt3d), cvc3ddot1/4(ilt3d), Lilt3ddot/1(ilt3d), ilt3d-/1
  iacd/1 -> cvc0ddot/7(iacd)

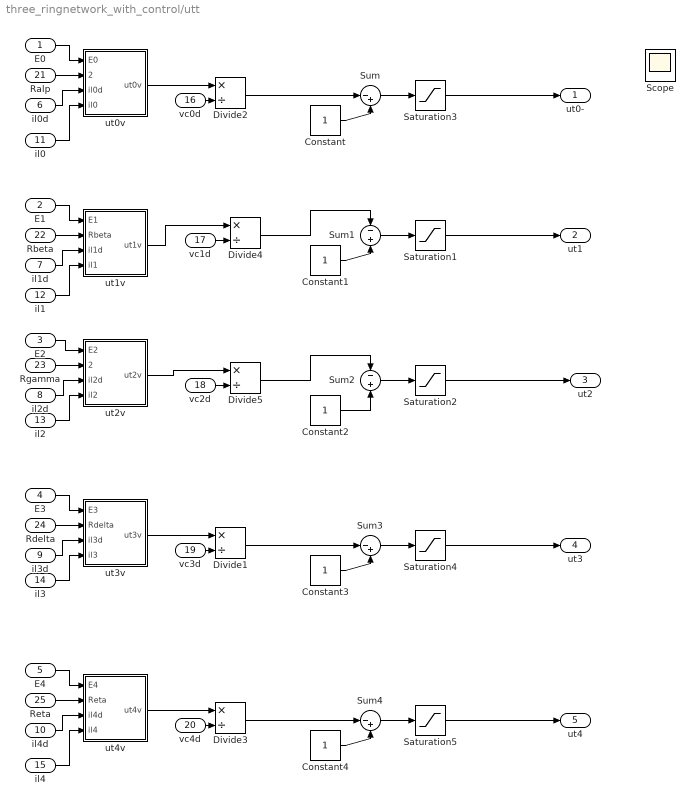
== system three_ringnetwork_with_control/utt ==
  E0 : Inport
  E1 : Inport  Port=2
  E2 : Inport  Port=3
  E3 : Inport  Port=4
  E4 : Inport  Port=5
  il0d : Inport  Port=6
  il1d : Inport  Port=7
  il2d : Inport  Port=8
  il3d : Inport  Port=9
  il4d : Inport  Port=10
  il0 : Inport  Port=11
  il1 : Inport  Port=12
  il2 : Inport  Port=13
  il3 : Inport  Port=14
  il4 : Inport  Port=15
  vc0d : Inport  Port=16
  vc1d : Inport  Port=17
  vc2d : Inport  Port=18
  vc3d : Inport  Port=19
  vc4d : Inport  Port=20
  Ralp : Inport  Port=21
  Rbeta : Inport  Port=22
  Rgamma : Inport  Port=23
  Rdelta : Inport  Port=24
  Reta : Inport  Port=25
  Constant{,1..4} (5 alike) : Constant
  Divide{1..5} (5 alike) : Product  Inputs=*/
  Saturation{1..5} (5 alike) : Saturate  UpperLimit=1  LowerLimit=0
  Scope : Scope
  Sum : Sum  Inputs=|-+
  Sum1 : Sum  Inputs=-+
  Sum2 : Sum  Inputs=-+
  Sum3 : Sum  Inputs=|-+
  Sum4 : Sum  Inputs=|-+
  ut0v : MATLAB Function  TreatAsAtomicUnit=on
  ut1v : MATLAB Function  TreatAsAtomicUnit=on
  ut2v : MATLAB Function  TreatAsAtomicUnit=on
  ut3v : MATLAB Function  TreatAsAtomicUnit=on
  ut4v : MATLAB Function  TreatAsAtomicUnit=on
  ut0- : Outport
  ut1 : Outport  Port=2
  ut2 : Outport  Port=3
  ut3 : Outport  Port=4
  ut4 : Outport  Port=5
  wires:
  vc0d/1 -> Divide2/2
  vc1d/1 -> Divide4/2
  vc2d/1 -> Divide5/2
  ut1v/1(ut1v) -> Divide4/1
  ut0v/1(ut0v) -> Divide2/1
  Divide2/1 -> Sum/1
  Sum/1 -> Saturation3/1
  Constant/1 -> Sum/2
  Constant1/1 -> Sum1/2
  Sum1/1 -> Saturation1/1
  ut2v/1(ut2v) -> Divide5/1
  Constant2/1 -> Sum2/2
  Sum2/1 -> Saturation2/1
  il2/1 -> ut2v/4(il2)
  il2d/1 -> ut2v/3(il2d)
  Rgamma/1 -> ut2v/2(Rgamma)
  E2/1 -> ut2v/1(E2)
  il1/1 -> ut1v/4(il1)
  il1d/1 -> ut1v/3(il1d)
  Rbeta/1 -> ut1v/2(Rbeta)
  E1/1 -> ut1v/1(E1)
  il0/1 -> ut0v/4(il0)
  il0d/1 -> ut0v/3(il0d)
  Ralp/1 -> ut0v/2(Ralpha)
  E0/1 -> ut0v/1(E0)
  Divide4/1 -> Sum1/1
  Divide5/1 -> Sum2/1
  Saturation2/1 -> ut2/1
  Saturation1/1 -> ut1/1
  Saturation3/1 -> ut0-/1
  vc3d/1 -> Divide1/2
  ut3v/1(ut3v) -> Divide1/1
  Divide1/1 -> Sum3/1
  Sum3/1 -> Saturation4/1
  Constant3/1 -> Sum3/2
  il3/1 -> ut3v/4(il3)
  il3d/1 -> ut3v/3(il3d)
  Rdelta/1 -> ut3v/2(Rdelta)
  E3/1 -> ut3v/1(E3)
  Saturation4/1 -> ut3/1
  vc4d/1 -> Divide3/2
  ut4v/1(ut4v) -> Divide3/1
  Divide3/1 -> Sum4/1
  Sum4/1 -> Saturation5/1
  Constant4/1 -> Sum4/2
  il4/1 -> ut4v/4(il4)
  il4d/1 -> ut4v/3(il4d)
  Reta/1 -> ut4v/2(Reta)
  E4/1 -> ut4v/1(E4)
  Saturation5/1 -> ut4/1

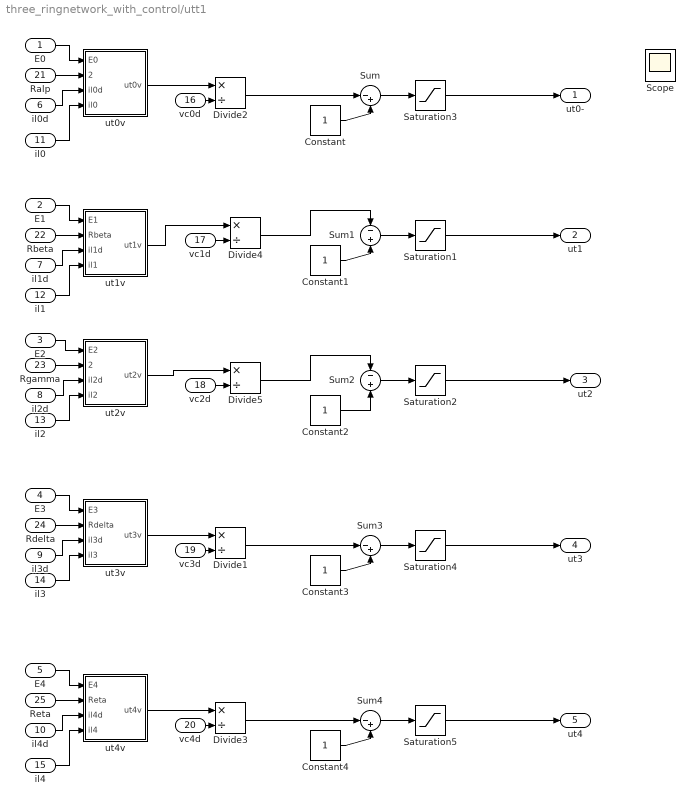
== system three_ringnetwork_with_control/utt1 ==
  E0 : Inport
  E1 : Inport  Port=2
  E2 : Inport  Port=3
  E3 : Inport  Port=4
  E4 : Inport  Port=5
  il0d : Inport  Port=6
  il1d : Inport  Port=7
  il2d : Inport  Port=8
  il3d : Inport  Port=9
  il4d : Inport  Port=10
  il0 : Inport  Port=11
  il1 : Inport  Port=12
  il2 : Inport  Port=13
  il3 : Inport  Port=14
  il4 : Inport  Port=15
  vc0d : Inport  Port=16
  vc1d : Inport  Port=17
  vc2d : Inport  Port=18
  vc3d : Inport  Port=19
  vc4d : Inport  Port=20
  Ralp : Inport  Port=21
  Rbeta : Inport  Port=22
  Rgamma : Inport  Port=23
  Rdelta : Inport  Port=24
  Reta : Inport  Port=25
  Constant{,1..4} (5 alike) : Constant
  Divide{1..5} (5 alike) : Product  Inputs=*/
  Saturation{1..5} (5 alike) : Saturate  UpperLimit=1  LowerLimit=0
  Scope : Scope
  Sum : Sum  Inputs=|-+
  Sum1 : Sum  Inputs=-+
  Sum2 : Sum  Inputs=-+
  Sum3 : Sum  Inputs=|-+
  Sum4 : Sum  Inputs=|-+
  ut0v : MATLAB Function  TreatAsAtomicUnit=on
  ut1v : MATLAB Function  TreatAsAtomicUnit=on
  ut2v : MATLAB Function  TreatAsAtomicUnit=on
  ut3v : MATLAB Function  TreatAsAtomicUnit=on
  ut4v : MATLAB Function  TreatAsAtomicUnit=on
  ut0- : Outport
  ut1 : Outport  Port=2
  ut2 : Outport  Port=3
  ut3 : Outport  Port=4
  ut4 : Outport  Port=5
  wires:
  vc0d/1 -> Divide2/2
  vc1d/1 -> Divide4/2
  vc2d/1 -> Divide5/2
  ut1v/1(ut1v) -> Divide4/1
  ut0v/1(ut0v) -> Divide2/1
  Divide2/1 -> Sum/1
  Sum/1 -> Saturation3/1
  Constant/1 -> Sum/2
  Constant1/1 -> Sum1/2
  Sum1/1 -> Saturation1/1
  ut2v/1(ut2v) -> Divide5/1
  Constant2/1 -> Sum2/2
  Sum2/1 -> Saturation2/1
  il2/1 -> ut2v/4(il2)
  il2d/1 -> ut2v/3(il2d)
  Rgamma/1 -> ut2v/2(Rgamma)
  E2/1 -> ut2v/1(E2)
  il1/1 -> ut1v/4(il1)
  il1d/1 -> ut1v/3(il1d)
  Rbeta/1 -> ut1v/2(Rbeta)
  E1/1 -> ut1v/1(E1)
  il0/1 -> ut0v/4(il0)
  il0d/1 -> ut0v/3(il0d)
  Ralp/1 -> ut0v/2(Ralpha)
  E0/1 -> ut0v/1(E0)
  Divide4/1 -> Sum1/1
  Divide5/1 -> Sum2/1
  Saturation2/1 -> ut2/1
  Saturation1/1 -> ut1/1
  Saturation3/1 -> ut0-/1
  vc3d/1 -> Divide1/2
  ut3v/1(ut3v) -> Divide1/1
  Divide1/1 -> Sum3/1
  Sum3/1 -> Saturation4/1
  Constant3/1 -> Sum3/2
  il3/1 -> ut3v/4(il3)
  il3d/1 -> ut3v/3(il3d)
  Rdelta/1 -> ut3v/2(Rdelta)
  E3/1 -> ut3v/1(E3)
  Saturation4/1 -> ut3/1
  vc4d/1 -> Divide3/2
  ut4v/1(ut4v) -> Divide3/1
  Divide3/1 -> Sum4/1
  Sum4/1 -> Saturation5/1
  Constant4/1 -> Sum4/2
  il4/1 -> ut4v/4(il4)
  il4d/1 -> ut4v/3(il4d)
  Reta/1 -> ut4v/2(Reta)
  E4/1 -> ut4v/1(E4)
  Saturation5/1 -> ut4/1

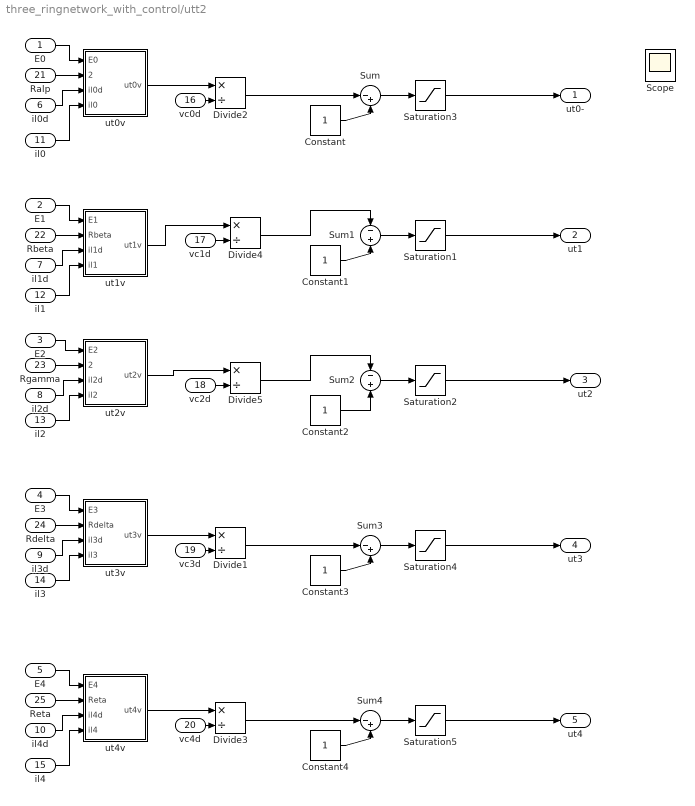
== system three_ringnetwork_with_control/utt2 ==
  E0 : Inport
  E1 : Inport  Port=2
  E2 : Inport  Port=3
  E3 : Inport  Port=4
  E4 : Inport  Port=5
  il0d : Inport  Port=6
  il1d : Inport  Port=7
  il2d : Inport  Port=8
  il3d : Inport  Port=9
  il4d : Inport  Port=10
  il0 : Inport  Port=11
  il1 : Inport  Port=12
  il2 : Inport  Port=13
  il3 : Inport  Port=14
  il4 : Inport  Port=15
  vc0d : Inport  Port=16
  vc1d : Inport  Port=17
  vc2d : Inport  Port=18
  vc3d : Inport  Port=19
  vc4d : Inport  Port=20
  Ralp : Inport  Port=21
  Rbeta : Inport  Port=22
  Rgamma : Inport  Port=23
  Rdelta : Inport  Port=24
  Reta : Inport  Port=25
  Constant{,1..4} (5 alike) : Constant
  Divide{1..5} (5 alike) : Product  Inputs=*/
  Saturation{1..2,4..5} (4 alike) : Saturate  UpperLimit=1  LowerLimit=0
  Saturation3 : Saturate  UpperLimit=1  LowerLimit=0  ZeroCross=off
  Scope : Scope
  Sum : Sum  Inputs=|-+
  Sum1 : Sum  Inputs=-+
  Sum2 : Sum  Inputs=-+
  Sum3 : Sum  Inputs=|-+
  Sum4 : Sum  Inputs=|-+
  ut0v : MATLAB Function  TreatAsAtomicUnit=on
  ut1v : MATLAB Function  TreatAsAtomicUnit=on
  ut2v : MATLAB Function  TreatAsAtomicUnit=on
  ut3v : MATLAB Function  TreatAsAtomicUnit=on
  ut4v : MATLAB Function  TreatAsAtomicUnit=on
  ut0- : Outport
  ut1 : Outport  Port=2
  ut2 : Outport  Port=3
  ut3 : Outport  Port=4
  ut4 : Outport  Port=5
  wires:
  vc0d/1 -> Divide2/2
  vc1d/1 -> Divide4/2
  vc2d/1 -> Divide5/2
  ut1v/1(ut1v) -> Divide4/1
  ut0v/1(ut0v) -> Divide2/1
  Divide2/1 -> Sum/1
  Sum/1 -> Saturation3/1
  Constant/1 -> Sum/2
  Constant1/1 -> Sum1/2
  Sum1/1 -> Saturation1/1
  ut2v/1(ut2v) -> Divide5/1
  Constant2/1 -> Sum2/2
  Sum2/1 -> Saturation2/1
  il2/1 -> ut2v/4(il2)
  il2d/1 -> ut2v/3(il2d)
  Rgamma/1 -> ut2v/2(Rgamma)
  E2/1 -> ut2v/1(E2)
  il1/1 -> ut1v/4(il1)
  il1d/1 -> ut1v/3(il1d)
  Rbeta/1 -> ut1v/2(Rbeta)
  E1/1 -> ut1v/1(E1)
  il0/1 -> ut0v/4(il0)
  il0d/1 -> ut0v/3(il0d)
  Ralp/1 -> ut0v/2(Ralpha)
  E0/1 -> ut0v/1(E0)
  Divide4/1 -> Sum1/1
  Divide5/1 -> Sum2/1
  Saturation2/1 -> ut2/1
  Saturation1/1 -> ut1/1
  Saturation3/1 -> ut0-/1
  vc3d/1 -> Divide1/2
  ut3v/1(ut3v) -> Divide1/1
  Divide1/1 -> Sum3/1
  Sum3/1 -> Saturation4/1
  Constant3/1 -> Sum3/2
  il3/1 -> ut3v/4(il3)
  il3d/1 -> ut3v/3(il3d)
  Rdelta/1 -> ut3v/2(Rdelta)
  E3/1 -> ut3v/1(E3)
  Saturation4/1 -> ut3/1
  vc4d/1 -> Divide3/2
  ut4v/1(ut4v) -> Divide3/1
  Divide3/1 -> Sum4/1
  Sum4/1 -> Saturation5/1
  Constant4/1 -> Sum4/2
  il4/1 -> ut4v/4(il4)
  il4d/1 -> ut4v/3(il4d)
  Reta/1 -> ut4v/2(Reta)
  E4/1 -> ut4v/1(E4)
  Saturation5/1 -> ut4/1

== matlab function three_ringnetwork_with_control/whole_sys1 ==
  data: u0 input; u1 input; u2 input; u3 input; u4 input; E0 input; E1 input; E2 input; E3 input; E4 input; R1t0 input; R1t1 input; R1t2 input; R1t3 input; R1t4 input; R2t0 input; R2t1 input; R2t2 input; R2t3 input; R2t4 input; C0 input; C1 input; C2 input; C3 input; C4 input; L0 input; L1 input; L2 input; L3 input; L4 input; Lt0 input; Lt1 input; Lt2 input; Lt3 input; Lt4 input; il0d input; il1d input; il2d input; il3d input; il4d input; il0 input; il1 input; il2 input; il3 input; il4 input; vc0 input; vc1 input; vc2 input; vc3 input; vc4 input; ilt0 input; ilt1 input; ilt2 input; ilt3 input; ilt4 input; iab input; vc0d input; vc1d input; vc2d input; vc3d input; vc4d input; ilt0d input; ilt1d input; ilt2d input; ilt3d input; ilt4d input; il0dot output; il1dot output; il2dot output; il3dot output; il4dot output; vc0dot output; vc1dot output; vc2dot output; vc3dot output; vc4dot output; ilt0dot output; ilt1dot output; ilt2dot output; ilt3dot output; ilt4dot output; He0 output; He1 output; He2 output; He3 output; He4 output; He output; H output; H0 output; H1 output; H2 output; H3 output; H4 output; itot output; unused input
function [il0dot,il1dot,il2dot,il3dot, il4dot,vc0dot,vc1dot,vc2dot,vc3dot,vc4dot,ilt0dot,ilt1dot,ilt2dot,ilt3dot,ilt4dot,He0,He1,He2,He3,He4,He,H,H0,H1,H2,H3,H4,itot]= fcn(u0,u1,u2,u3,u4,E0,E1,E2,E3,E4,R1t0,R1t1,R1t2,R1t3,R1t4,R2t0,R2t1,R2t2,R2t3,R2t4,C0,C1,C2,C3,C4,L0,L1,L2,L3,L4,Lt0,Lt1,Lt2,Lt3,Lt4,il0d,il1d,il2d,il3d,il4d,il0,il1,il2,il3,il4,vc0,vc1,vc2,vc3,vc4,ilt0,ilt1,ilt2,ilt3,ilt4,iab,vc0d,vc1d,vc2d,vc3d,vc4d,ilt0d,ilt1d,ilt2d,ilt3d,ilt4d,~)



il0dot=((-(1-u0)*vc0)+E0)/L0;
il1dot=((-(1-u1)*vc1)+E1)/L1;
il2dot=((-(1-u2)*vc2)+E2)/L2;
il3dot=((-(1-u3)*vc3)+E3)/L3;
il4dot=((-(1-u4)*vc4)+E4)/L4;


vc0dot=(((1-u0)*il0)-ilt0+ilt4-(vc0/R2t4)+iab)/C0;
vc1dot=(((1-u1)*il1)-ilt1+ilt0-(vc1/R2t0))/C1;
vc2dot=(((1-u2)*il2)-ilt2+ilt1-(vc2/R2t1))/C2;
vc3dot=(((1-u3)*il3)-ilt3+ilt2-(vc3/R2t2))/C3;
vc4dot=(((1-u4)*il4)-ilt4+ilt3-(vc4/R2t3))/C4;


ilt0dot=(vc0-vc1-(R1t0*ilt0))/Lt0;
ilt1dot=(vc1-vc2-(R1t1*ilt1))/Lt1;
ilt2dot=(vc2-vc3-(R1t2*ilt2))/Lt2;
ilt3dot=(vc3-vc4-(R1t3*ilt3))/Lt3;
ilt4dot=(vc4-vc0-(R1t4*ilt4))/Lt4;

%iabdot=(vc0-vcb-(Rab*iab))/Lab;

itot=ilt0+ilt1+ilt2+ilt3+ilt4;

H0 =0.5*((L0*(il0^2))+(C0*(vc0^2))+(Lt0*(ilt0^2)));
H1 =0.5*((L1*(il1^2))+(C1*(vc1^2))+(Lt1*(ilt1^2)));
H2 =0.5*((L2*(il2^2))+(C2*(vc2^2))+(Lt2*(ilt2^2)));
H3 =0.5*((L3*(il3^2))+(C3*(vc3^2))+(Lt3*(ilt3^2)));
H4 =0.5*((L4*(il4^2))+(C4*(vc4^2))+(Lt4*(ilt4^2)));

He0=0.5*((L0*((il0-il0d)^2))+(C0*((vc0-vc0d)^2))+(Lt0*((ilt0-ilt0d)^2)));
He1=0.5*((L1*((il1-il1d)^2))+(C1*((vc1-vc1d)^2))+(Lt1*((ilt1-ilt1d)^2)));
He2=0.5*((L2*((il2-il2d)^2))+(C2*((vc2-vc2d)^2))+(Lt2*((ilt2-ilt2d)^2)));
He3=0.5*((L3*((il3-il3d)^2))+(C3*((vc3-vc3d)^2))+(Lt3*((ilt3-ilt3d)^2)));
He4=0.5*((L4*((il4-il4d)^2))+(C4*((vc4-vc4d)^2))+(Lt4*((ilt4-ilt4d)^2)));
H=H0+H2+H2+H3+H4;
He=He0+He1+He2+He3+He4;
%He=0.5*((L0*(il0-il0d)^2)+(C0*(vc0-vc0d)^2)+(Lt0*(ilt0-ilt0d)^2)+(L1*(il1-il1d)^2)+(C1*(vc1-vc1d)^2)+(Lt1*(ilt1-ilt1d)^2)+(L2*(il2-il2d)^2)+(C2*(vc2-vc2d)^2)+(Lt2*(ilt2-ilt2d)^2));

== matlab function three_ringnetwork_with_control/whole_sys ==
  data: u0 input; u1 input; u2 input; u3 input; u4 input; E0 input; E1 input; E2 input; E3 input; E4 input; R1t0 input; R1t1 input; R1t2 input; R1t3 input; R1t4 input; R2t0 input; R2t1 input; R2t2 input; R2t3 input; R2t4 input; C0 input; C1 input; C2 input; C3 input; C4 input; L0 input; L1 input; L2 input; L3 input; L4 input; Lt0 input; Lt1 input; Lt2 input; Lt3 input; Lt4 input; il0d input; il1d input; il2d input; il3d input; il4d input; Rab input; Lab input; Rac input; Lac input; il0 input; il1 input; il2 input; il3 input; il4 input; vc0 input; vc1 input; vc2 input; vc3 input; vc4 input; ilt0 input; ilt1 input; ilt2 input; ilt3 input; ilt4 input; iab input; iac input; vc0b input; vc0c input; vc0d input; vc1d input; vc2d input; vc3d input; vc4d input; ilt0d input; ilt1d input; ilt2d input; ilt3d input; ilt4d input; il0dot output; il1dot output; il2dot output; il3dot output; il4dot output; vc0dot output; vc1dot output; vc2dot output; vc3dot output; vc4dot output; ilt0dot output; ilt1dot output; ilt2dot output; ilt3dot output; ilt4dot output; iabdot output; iacdot output; He0 output; He1 output; He2 output; He3 output; He4 output; He output; H output; H0 output; H1 output; H2 output; H3 output; H4 output; iabd input; iacd input
function [il0dot,il1dot,il2dot,il3dot, il4dot,vc0dot,vc1dot,vc2dot,vc3dot,vc4dot,ilt0dot,ilt1dot,ilt2dot,ilt3dot,ilt4dot,iabdot,iacdot,He0,He1,He2,He3,He4,He,H,H0,H1,H2,H3,H4]= fcn(u0,u1,u2,u3,u4,E0,E1,E2,E3,E4,R1t0,R1t1,R1t2,R1t3,R1t4,R2t0,R2t1,R2t2,R2t3,R2t4,C0,C1,C2,C3,C4,L0,L1,L2,L3,L4,Lt0,Lt1,Lt2,Lt3,Lt4, il0d,il1d,il2d,il3d,il4d,Rab, Lab,Rac,Lac,il0,il1,il2,il3,il4,vc0,vc1,vc2,vc3,vc4,ilt0,ilt1,ilt2,ilt3,ilt4,iab,iac,vc0b,vc0c,vc0d,vc1d,vc2d,vc3d,vc4d,ilt0d,ilt1d,ilt2d,ilt3d,ilt4d,iabd,iacd)



il0dot=((-(1-u0)*vc0)+E0)/L0;
il1dot=((-(1-u1)*vc1)+E1)/L1;
il2dot=((-(1-u2)*vc2)+E2)/L2;
il3dot=((-(1-u3)*vc3)+E3)/L3;
il4dot=((-(1-u4)*vc4)+E4)/L4;


vc0dot=(((1-u0)*il0)-ilt0+ilt4-(vc0/R2t4)-iab)/C0;
vc1dot=(((1-u1)*il1)-ilt1+ilt0-(vc1/R2t0)-iac)/C1;
vc2dot=(((1-u2)*il2)-ilt2+ilt1-(vc2/R2t1))/C2;
vc3dot=(((1-u3)*il3)-ilt3+ilt2-(vc3/R2t2))/C3;
vc4dot=(((1-u4)*il4)-ilt4+ilt3-(vc4/R2t3))/C4;


ilt0dot=(vc0-vc1-(R1t0*ilt0))/Lt0;
ilt1dot=(vc1-vc2-(R1t1*ilt1))/Lt1;
ilt2dot=(vc2-vc3-(R1t2*ilt2))/Lt2;
ilt3dot=(vc3-vc4-(R1t3*ilt3))/Lt3;
ilt4dot=(vc4-vc0-(R1t4*ilt4))/Lt4;

iabdot= (-Rab*iab+vc0-vc0b)/Lab;
iacdot= (-Rac*iac+vc1-vc0c)/Lac;

%itot=R2t0*vc0dot*(ilt0-ilt4)+R2t1*vc1dot*(ilt1-ilt0)+R2t2*vc2dot*(ilt2-ilt1)+R2t3*vc3dot*(ilt3-ilt2)+R2t4*vc4dot*(ilt4-ilt3);

%itot=ilt0+ilt1+ilt2+ilt3+ilt4;
% w0=0.6737;
% A0=17;
% Ub=((-A0*(w0^2)/vc0)*sin(w0*t/(sqrt(Lb*Cb))))+(sqrt(Lb/Cb)*A0/(vc0*Rb))*cos(w0*t/(sqrt(Lb*Cb)))+(A0/vc0)*sin(w0*t/(sqrt(Lb*Cb)));
% vcbss=A0*sin((w0/(sqrt(Lb*Cb)))*t);
% ilbd= Cb*A0*w0*(1/sqrt(Lb*Cb))*cos((w0/(sqrt(Lb*Cb)))*t)+(vcbss/Rb);

H0 =0.5*((L0*(il0^2))+(C0*(vc0^2))+(Lt0*(ilt0^2))+(Lab*(iab^2)));
H1 =0.5*((L1*(il1^2))+(C1*(vc1^2))+(Lt1*(ilt1^2))+(Lac*(iac^2)));
H2 =0.5*((L2*(il2^2))+(C2*(vc2^2))+(Lt2*(ilt2^2)));
H3 =0.5*((L3*(il3^2))+(C3*(vc3^2))+(Lt3*(ilt3^2)));
H4 =0.5*((L4*(il4^2))+(C4*(vc4^2))+(Lt4*(ilt4^2)));
% H_inv=0.5*((Lb*(ilb)^2)+(Cb*(vcb)^2));
% 
He0=0.5*((L0*((il0-il0d)^2))+(C0*((vc0-vc0d)^2))+(Lt0*((ilt0-ilt0d)^2))+(Lab*(iab-iabd)));
He1=0.5*((L1*((il1-il1d)^2))+(C1*((vc1-vc1d)^2))+(Lt1*((ilt1-ilt1d)^2))+(Lac*(iac-iacd)));
He2=0.5*((L2*((il2-il2d)^2))+(C2*((vc2-vc2d)^2))+(Lt2*((ilt2-ilt2d)^2)));
He3=0.5*((L3*((il3-il3d)^2))+(C3*((vc3-vc3d)^2))+(Lt3*((ilt3-ilt3d)^2)));
He4=0.5*((L4*((il4-il4d)^2))+(C4*((vc4-vc4d)^2))+(Lt4*((ilt4-ilt4d)^2)));
%He_inv=0.5*((Lb*(ilb-ilbd)^2)+(Cb*(vcb-vcbd)^2));
 H=H0+H1+H2+H3+H4;
 He=He0+He1+He2+He3+He4;
%H=0.5*((L0*(il0^2))+(C0*(vc0^2))+(Lt0*(ilt0^2))+(L1*(il1^2))+(C1*(vc1^2))+(Lt1*(ilt1^2))+(L2*(il2^2))+(C2*(vc2^2))+(Lt2*(ilt2^2)));
%He=0.5*((L0*(il0-il0d)^2)+(C0*(vc0-vc0d)^2)+(Lt0*(ilt0-ilt0d)^2)+(L1*(il1-il1d)^2)+(C1*(vc1-vc1d)^2)+(Lt1*(ilt1-ilt1d)^2)+(L2*(il2-il2d)^2)+(C2*(vc2-vc2d)^2)+(Lt2*(ilt2-ilt2d)^2));

== matlab function three_ringnetwork_with_control/whole_sys2 ==
  data: u0 input; u1 input; u2 input; u3 input; u4 input; E0 input; E1 input; E2 input; E3 input; E4 input; R1t0 input; R1t1 input; R1t2 input; R1t3 input; R1t4 input; R2t0 input; R2t1 input; R2t2 input; R2t3 input; R2t4 input; C0 input; C1 input; C2 input; C3 input; C4 input; L0 input; L1 input; L2 input; L3 input; L4 input; Lt0 input; Lt1 input; Lt2 input; Lt3 input; Lt4 input; il0d input; il1d input; il2d input; il3d input; il4d input; il0 input; il1 input; il2 input; il3 input; il4 input; vc0 input; vc1 input; vc2 input; vc3 input; vc4 input; ilt0 input; ilt1 input; ilt2 input; ilt3 input; ilt4 input; iac input; vc0d input; vc1d input; vc2d input; vc3d input; vc4d input; ilt0d input; ilt1d input; ilt2d input; ilt3d input; ilt4d input; il0dot output; il1dot output; il2dot output; il3dot output; il4dot output; vc0dot output; vc1dot output; vc2dot output; vc3dot output; vc4dot output; ilt0dot output; ilt1dot output; ilt2dot output; ilt3dot output; ilt4dot output; He0 output; He1 output; He2 output; He3 output; He4 output; He output; H output; H0 output; H1 output; H2 output; H3 output; H4 output; itot output
function [il0dot,il1dot,il2dot,il3dot, il4dot,vc0dot,vc1dot,vc2dot,vc3dot,vc4dot,ilt0dot,ilt1dot,ilt2dot,ilt3dot,ilt4dot,He0,He1,He2,He3,He4,He,H,H0,H1,H2,H3,H4,itot]= fcn(u0,u1,u2,u3,u4,E0,E1,E2,E3,E4,R1t0,R1t1,R1t2,R1t3,R1t4,R2t0,R2t1,R2t2,R2t3,R2t4,C0,C1,C2,C3,C4,L0,L1,L2,L3,L4,Lt0,Lt1,Lt2,Lt3,Lt4,il0d,il1d,il2d,il3d,il4d,il0,il1,il2,il3,il4,vc0,vc1,vc2,vc3,vc4,ilt0,ilt1,ilt2,ilt3,ilt4,iac,vc0d,vc1d,vc2d,vc3d,vc4d,ilt0d,ilt1d,ilt2d,ilt3d,ilt4d)



il0dot=((-(1-u0)*vc0)+E0)/L0;
il1dot=((-(1-u1)*vc1)+E1)/L1;
il2dot=((-(1-u2)*vc2)+E2)/L2;
il3dot=((-(1-u3)*vc3)+E3)/L3;
il4dot=((-(1-u4)*vc4)+E4)/L4;


vc0dot=(((1-u0)*il0)-ilt0+ilt4-(vc0/R2t4)+iac)/C0;
vc1dot=(((1-u1)*il1)-ilt1+ilt0-(vc1/R2t0))/C1;
vc2dot=(((1-u2)*il2)-ilt2+ilt1-(vc2/R2t1))/C2;
vc3dot=(((1-u3)*il3)-ilt3+ilt2-(vc3/R2t2))/C3;
vc4dot=(((1-u4)*il4)-ilt4+ilt3-(vc4/R2t3))/C4;


ilt0dot=(vc0-vc1-(R1t0*ilt0))/Lt0;
ilt1dot=(vc1-vc2-(R1t1*ilt1))/Lt1;
ilt2dot=(vc2-vc3-(R1t2*ilt2))/Lt2;
ilt3dot=(vc3-vc4-(R1t3*ilt3))/Lt3;
ilt4dot=(vc4-vc0-(R1t4*ilt4))/Lt4;

itot=ilt0+ilt1+ilt2+ilt3+ilt4;

H0 =0.5*((L0*(il0^2))+(C0*(vc0^2))+(Lt0*(ilt0^2)));
H1 =0.5*((L1*(il1^2))+(C1*(vc1^2))+(Lt1*(ilt1^2)));
H2 =0.5*((L2*(il2^2))+(C2*(vc2^2))+(Lt2*(ilt2^2)));
H3 =0.5*((L3*(il3^2))+(C3*(vc3^2))+(Lt3*(ilt3^2)));
H4 =0.5*((L4*(il4^2))+(C4*(vc4^2))+(Lt4*(ilt4^2)));

He0=0.5*((L0*((il0-il0d)^2))+(C0*((vc0-vc0d)^2))+(Lt0*((ilt0-ilt0d)^2)));
He1=0.5*((L1*((il1-il1d)^2))+(C1*((vc1-vc1d)^2))+(Lt1*((ilt1-ilt1d)^2)));
He2=0.5*((L2*((il2-il2d)^2))+(C2*((vc2-vc2d)^2))+(Lt2*((ilt2-ilt2d)^2)));
He3=0.5*((L3*((il3-il3d)^2))+(C3*((vc3-vc3d)^2))+(Lt3*((ilt3-ilt3d)^2)));
He4=0.5*((L4*((il4-il4d)^2))+(C4*((vc4-vc4d)^2))+(Lt4*((ilt4-ilt4d)^2)));
H=H0+H2+H2+H3+H4;
He=He0+He1+He2+He3+He4;
%He=0.5*((L0*(il0-il0d)^2)+(C0*(vc0-vc0d)^2)+(Lt0*(ilt0-ilt0d)^2)+(L1*(il1-il1d)^2)+(C1*(vc1-vc1d)^2)+(Lt1*(ilt1-ilt1d)^2)+(L2*(il2-il2d)^2)+(C2*(vc2-vc2d)^2)+(Lt2*(ilt2-ilt2d)^2));
